simulink model "acik_cevrim_modeli"  (R2020b)
settings: Solver=VariableStepAuto  StartTime=0.0  StopTime=20  RelTol=1e-3
settings Model: Creator=amnessa  LastModifiedBy=amnessa

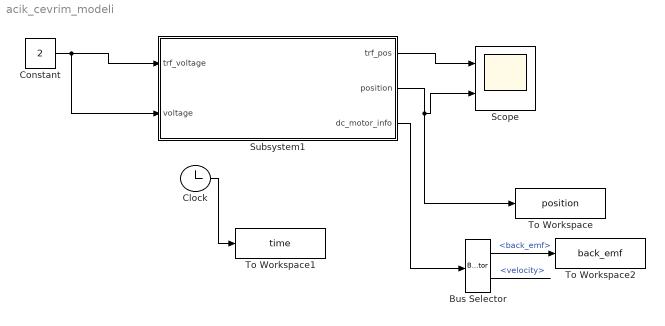
== system acik_cevrim_modeli ==
  Bus Selector : BusSelector  OutputSignals=back_emf,velocity
  Clock : Clock
  Constant : Constant  Value=2
  Scope : Scope  NumInputPorts=2
  Subsystem1 : Subsystem  mask{J=0.03, B=0.01, KT=0.5, R=8, L=0.45, KB=0.5}
      mask prompts: J "(J/KG*M^2)"; B "B(Nm/rad)"; KT "KT(NM/AMPER)"; R "R(OHM)"; L "L(H)"; KB "KB(Vsn/rad)"
  To Workspace : ToWorkspace  VariableName=position  SampleTime=-1
  To Workspace1 : ToWorkspace  VariableName=time  SampleTime=-1
  To Workspace2 : ToWorkspace  VariableName=back_emf  SampleTime=-1
  wires:
  Subsystem1/1(trf_pos) -> Scope/1
  Subsystem1/2(position) -> To Workspace/1, Scope/2
  Constant/1 -> Subsystem1/2(voltage), Subsystem1/1(trf_voltage)
  Clock/1 -> To Workspace1/1
  Subsystem1/3(dc_motor_info) -> Bus Selector/1
  Bus Selector/1 -> To Workspace2/1  "<back_emf>"
  Bus Selector/2 -> ?  "<velocity>"

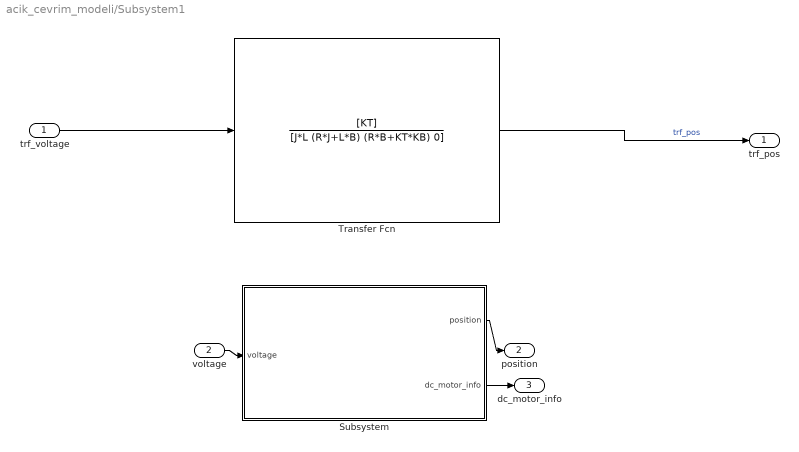
== system acik_cevrim_modeli/Subsystem1 ==
  trf_voltage : Inport
  voltage : Inport  Port=2
  Subsystem : Subsystem
  Transfer Fcn : TransferFcn  Numerator=[KT]  Denominator=[J*L (R*J+L*B) (R*B+KT*KB) 0]
  trf_pos : Outport
  position : Outport  Port=2
  dc_motor_info : Outport  Port=3
  wires:
  Transfer Fcn/1 -> trf_pos/1  "trf_pos"
  trf_voltage/1 -> Transfer Fcn/1
  Subsystem/1(position) -> position/1
  voltage/1 -> Subsystem/1(voltage)
  Subsystem/2(dc_motor_info) -> dc_motor_info/1

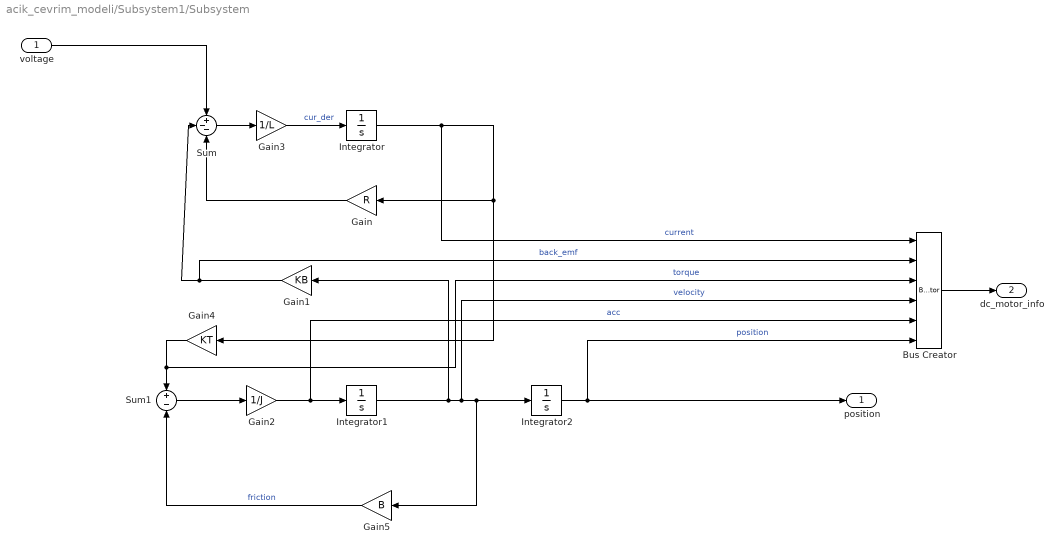
== system acik_cevrim_modeli/Subsystem1/Subsystem ==
  voltage : Inport
  Bus Creator : BusCreator  Inputs=6
  Gain : Gain  Gain=R
  Gain1 : Gain  Gain=KB
  Gain2 : Gain  Gain=1/J
  Gain3 : Gain  Gain=1/L
  Gain4 : Gain  Gain=KT
  Gain5 : Gain  Gain=B
  Integrator : Integrator
  Integrator1 : Integrator
  Integrator2 : Integrator
  Sum : Sum  Inputs=+--
  Sum1 : Sum  Inputs=+-
  position : Outport
  dc_motor_info : Outport  Port=2
  wires:
  Gain3/1 -> Integrator/1  "cur_der"
  Gain4/1 -> Bus Creator/3, Sum1/1  "torque"
  Integrator/1 -> Bus Creator/1, Gain4/1, Gain/1  "current"
  Gain2/1 -> Bus Creator/5, Integrator1/1  "acc"
  Integrator1/1 -> Gain1/1, Bus Creator/4, Gain5/1, Integrator2/1  "velocity"
  Sum1/1 -> Gain2/1
  Sum/1 -> Gain3/1
  Gain1/1 -> Bus Creator/2, Sum/2  "back_emf"
  Gain5/1 -> Sum1/2  "friction"
  Gain/1 -> Sum/3
  Integrator2/1 -> position/1, Bus Creator/6  "position"
  voltage/1 -> Sum/1
  Bus Creator/1 -> dc_motor_info/1
